simulink model "Hair_Health_Checker_Model"  (R2022a)
settings: Solver=VariableStepAuto  StartTime=0.0  StopTime=10.0  RelTol=1e-3
libraries: visionsources x2
settings Model: Creator=LENOVO  LastModifiedBy=LENOVO

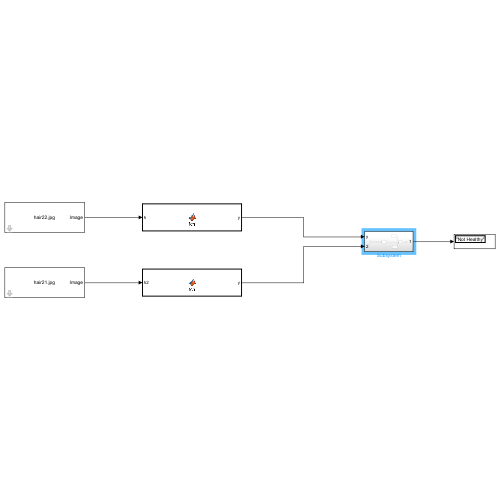
[thumbnail: Simulink's stored preview of the top-level diagram]
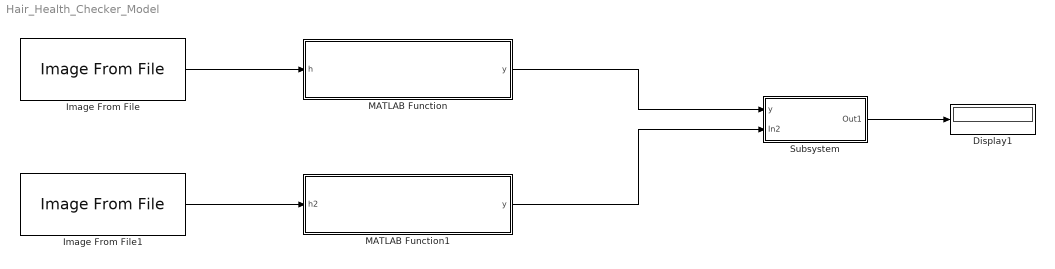
== system Hair_Health_Checker_Model ==
  Display1 : Display
  Image From File : visionsources/Image From File  Tag=vipblks_nd  FileName=C:\Users\LENOVO\OneDrive\Documents\L&T\MBD MATLAB\hair22.jpg  Ts=inf  imagePorts=One multidimensional signal  OutPortLabels=R|G|B  ImageDataType=Inherit from input image  sdImageDataType=uint(8)  Signed=on  WordLength=16  FractionLengthMode=User-defined  FractionLength=15
  Image From File1 : visionsources/Image From File  Tag=vipblks_nd  FileName=C:\Users\LENOVO\OneDrive\Documents\L&T\MBD MATLAB\hair21.jpg  Ts=inf  imagePorts=One multidimensional signal  OutPortLabels=R|G|B  ImageDataType=Inherit from input image  sdImageDataType=uint(8)  Signed=on  WordLength=16  FractionLengthMode=User-defined  FractionLength=15
  MATLAB Function : MATLAB Function  TreatAsAtomicUnit=on
  MATLAB Function1 : MATLAB Function  TreatAsAtomicUnit=on
  Subsystem : Subsystem
  wires:
  Image From File/1 -> MATLAB Function/1(h)
  Image From File1/1 -> MATLAB Function1/1(h2)
  MATLAB Function/1(y) -> Subsystem/1(y)
  MATLAB Function1/1(y) -> Subsystem/2(In2)
  Subsystem/1(Out1) -> Display1/1

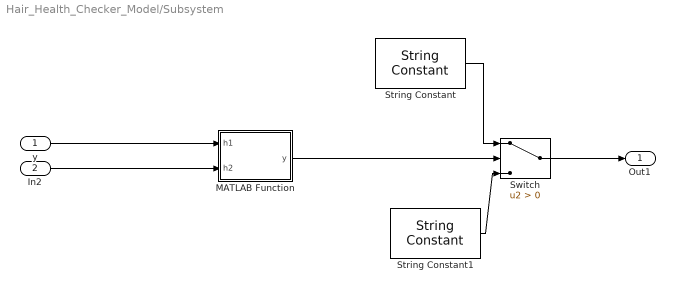
== system Hair_Health_Checker_Model/Subsystem ==
  y : Inport
  In2 : Inport  Port=2
  MATLAB Function : MATLAB Function  TreatAsAtomicUnit=on
  String Constant : StringConstant  String="\"Not Healthy\""
  String Constant1 : StringConstant  String="\"Healthy\""
  Switch : Switch  Criteria=u2 > Threshold  SaturateOnIntegerOverflow=off  InputSameDT=off
  Out1 : Outport
  wires:
  y/1 -> MATLAB Function/1(h1)
  In2/1 -> MATLAB Function/2(h2)
  Switch/1 -> Out1/1
  String Constant/1 -> Switch/1
  String Constant1/1 -> Switch/3
  MATLAB Function/1(y) -> Switch/2

== matlab function Hair_Health_Checker_Model/MATLAB Function ==
  data: h input; y output
function y = fcn(h)
h = imread('hair22.jpg');
%imshow(h)
[count,x] = imhist(h);
sz = size(h);
R = h(:,:,1);
%imshow(R)

%to grayscale
red=h(:,:,1);
green=h(:,:,2);
blue=h(:,:,3);
image_gray = im2gray(h);
% figure (1),subplot (3,3,2), imshow(image_gray), title('grayscale');

%tobinary
level = graythresh(image_gray);
BW = imbinarize (image_gray,level);
% figure(1),subplot(3,3,3),imshow(BW), title('binary');

%closing
se = strel('disk',10);
afterclosing = imclose(BW,se);
% figure(1), subplot (3,3,4), imshow(afterclosing), title('closing');

%opening
afteropen = imopen(afterclosing,se);
% figure(1), subplot (3,3,5),imshow(afteropen), title('opening');


y = level;
end

== matlab function Hair_Health_Checker_Model/Subsystem/MATLAB Function ==
  data: h1 input; y output; h2 input
function y = fcn(h1, h2)
if(h1>h2)
    y=1;
else
    y=0;
end

end

== matlab function Hair_Health_Checker_Model/MATLAB Function1 ==
  data: h2 input; y output
function y = fcn(h2)
h2 = imread('hair21.jpg');
%imshow(h2)
R2 = h2(:,:,1);
%imshow(R2)

%to grayscale
red2=h2(:,:,1);
green2=h2(:,:,2);
blue2=h2(:,:,3);
image_gray1 = im2gray(h2);
%figure (1),subplot (3,3,2), imshow(image_gray1), title('grayscale2');

%tobinary
level2 = graythresh(image_gray1);
BW2 = imbinarize (image_gray1,level2);
%figure(1),subplot(3,3,3),imshow(BW2), title('binary2');

%closing
se2 = strel('disk',10);
afterclosing2 = imclose(BW2,se2);
%figure(1), subplot (3,3,4), imshow(afterclosing2), title('closing2');

%opening
afteropen2 = imopen(afterclosing2 ,se2);
%figure(1), subplot (3,3,5),imshow(afteropen2), title('opening2');

y = level2;
